simulink library "ESTS_TFY_YawMomFromFx"  (R2023b)
settings: Solver=VariableStepAuto  StartTime=0.0  StopTime=10.0  RelTol=1e-3
settings Model: Creator=blatak  LastModifiedBy=blatak
settings ModelReferenceCC: EnableRefExpFcnMdlSchedulingChecks=on

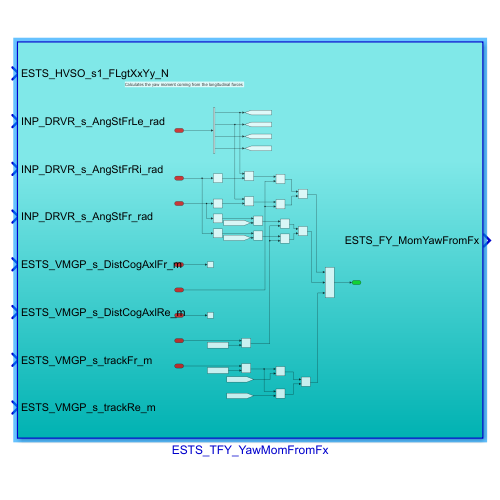
[thumbnail: Simulink's stored preview of the top-level diagram]
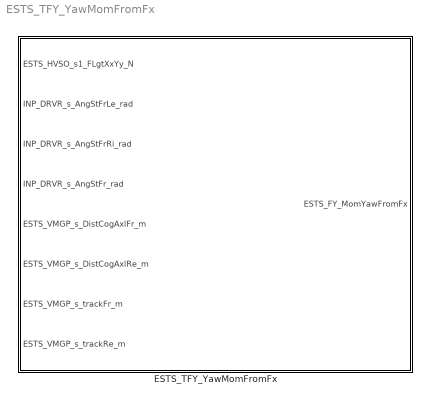
== system ESTS_TFY_YawMomFromFx ==
  ESTS_TFY_YawMomFromFx : Subsystem  Description=Calculates the yaw moment coming from the longitudinal forces

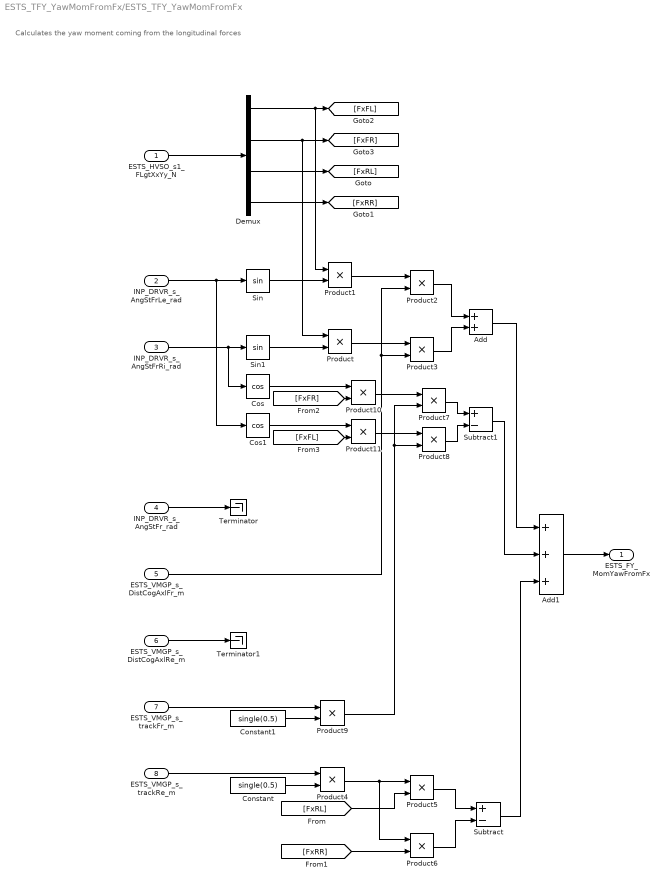
== system ESTS_TFY_YawMomFromFx/ESTS_TFY_YawMomFromFx ==
  note: Calculates the yaw moment coming from the longitudinal forces
  ESTS_HVSO_s1_FLgtXxYy_N : Inport  Description=Estimation of tyre longitudinal forces - vector
  INP_DRVR_s_AngStFrLe_rad : Inport  Description=Steering wheel angle FL - calculated only from steering ratio (Ackerman neglected now)  Port=2
  INP_DRVR_s_AngStFrRi_rad : Inport  Description=Steering wheel angle FR - calculated only from steering ratio (Ackerman neglected now)  Port=3
  INP_DRVR_s_AngStFr_rad : Inport  Description=|  Port=4
      | Steering wheel angle front - calculated as an average FL and FR,
      | used for single track model, later more sophisticated calculation method needed 
      | than only an average
  ESTS_VMGP_s_DistCogAxlFr_m : Inport  Description=X distance from front axle (wheel center) to cog  Port=5
  ESTS_VMGP_s_DistCogAxlRe_m : Inport  Description=X distance from rear axle (wheel center) to cog  Port=6
  ESTS_VMGP_s_trackFr_m : Inport  Description=|  Port=7
      | Front vehicle track - y-distance between tyre contact points left to right, front axle
      | in static position, no change due to kinematic in suspension movement
  ESTS_VMGP_s_trackRe_m : Inport  Description=|  Port=8
      | Rear vehicle track - y-distance between tyre contact points left to right, rear axle
      | in static position, no change due to kinematic in suspension movement
  Add : Sum
  Add1 : Sum  Inputs=+++
  Constant : Constant  Value=single(0.5)
  Constant1 : Constant  Value=single(0.5)
  Cos : Trigonometry  Operator=cos
  Cos1 : Trigonometry  Operator=cos
  Demux : Demux
  Product{,1..11} (12 alike) : Product
  Sin : Trigonometry
  Sin1 : Trigonometry
  Subtract : Sum  Inputs=+-
  Subtract1 : Sum  Inputs=+-
  Terminator : Terminator
  Terminator1 : Terminator
  ESTS_FY_MomYawFromFx : Outport  Description=Yaw moment coming from longitudinal forces
  wires:
  ESTS_HVSO_s1_FLgtXxYy_N/1 -> Demux/1
  INP_DRVR_s_AngStFrLe_rad/1 -> Sin/1, Cos1/1
  INP_DRVR_s_AngStFrRi_rad/1 -> Cos/1, Sin1/1
  Demux/2 -> [FxFR], Product/1
  Sin1/1 -> Product/2
  Sin/1 -> Product1/2
  Demux/1 -> [FxFL], Product1/1
  Product1/1 -> Product2/1
  ESTS_VMGP_s_DistCogAxlFr_m/1 -> Product3/2, Product2/2
  Product/1 -> Product3/1
  Product2/1 -> Add/1
  Product3/1 -> Add/2
  ESTS_VMGP_s_trackRe_m/1 -> Product4/1
  Constant/1 -> Product4/2
  Demux/3 -> [FxRL]
  Demux/4 -> [FxRR]
  Product4/1 -> Product6/1, Product5/1
  [FxRL] -> Product5/2
  [FxRR] -> Product6/2
  Product5/1 -> Subtract/1
  Product6/1 -> Subtract/2
  Cos/1 -> Product10/1
  Cos1/1 -> Product11/1
  Constant1/1 -> Product9/2
  ESTS_VMGP_s_trackFr_m/1 -> Product9/1
  Product9/1 -> Product8/2, Product7/2
  [FxFR] -> Product10/2
  [FxFL] -> Product11/2
  Product10/1 -> Product7/1
  Product11/1 -> Product8/1
  Product8/1 -> Subtract1/2
  Product7/1 -> Subtract1/1
  Add/1 -> Add1/1
  Subtract1/1 -> Add1/2
  Subtract/1 -> Add1/3
  Add1/1 -> ESTS_FY_MomYawFromFx/1
  INP_DRVR_s_AngStFr_rad/1 -> Terminator/1
  ESTS_VMGP_s_DistCogAxlRe_m/1 -> Terminator1/1
